simulink model "slau3"  (Simulink 9.1)
settings: Solver=ode45  StartTime=0.0  StopTime=5.0  RelTol=1e-3  EnableMultiTasking=on
settings Model: Creator=pustovskix.2018  LastModifiedBy=bukova.2018
settings DataIOCC: LimitDataPoints=on  SignalLoggingSaveFormat=ModelDataLogs
settings OptimizationCC: ExpressionDepthLimit=2147483647
settings DebuggingCC: SolverPrmCheckMsg=warning  FcnCallInpInsideContextMsg=warning  StateNameClashWarn=warning
settings GRTTargetCC: GeneratePreprocessorConditionals=Disable all

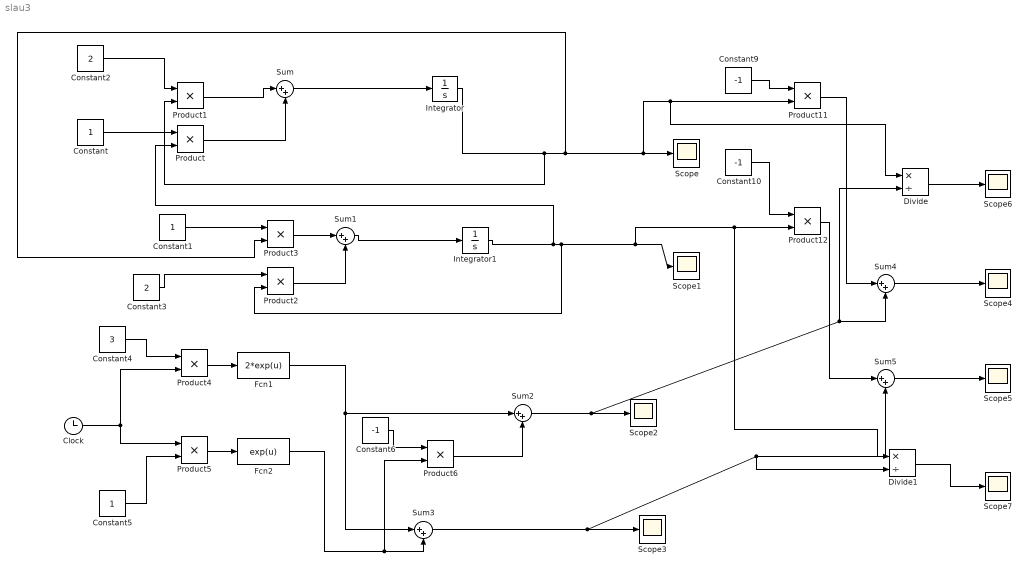
== system slau3 ==
  Clock : Clock
  Constant : Constant
  Constant1 : Constant
  Constant10 : Constant  Value=-1
  Constant2 : Constant  Value=2
  Constant3 : Constant  Value=2
  Constant4 : Constant  Value=3
  Constant5 : Constant
  Constant6 : Constant  Value=-1
  Constant9 : Constant  Value=-1
  Divide : Product  Inputs=*/
  Divide1 : Product  Inputs=*/
  Fcn1 : Fcn  Expr=2*exp(u)
  Fcn2 : Fcn  Expr=exp(u)
  Integrator : Integrator  InitialCondition=1
  Integrator1 : Integrator  InitialCondition=3
  Product{,1..6,11..12} (9 alike) : Product  RndMeth=Zero
  Scope{,1..7} (8 alike) : Scope
  Sum{,1..5} (6 alike) : Sum  Inputs=|++
  wires:
  Integrator1/1 -> Product2/2, Scope1/1, Divide1/1, Product12/2, Product/2
  Integrator/1 -> Product3/2, Scope/1, Divide/1, Product11/2, Product1/2
  Sum/1 -> Integrator/1
  Sum1/1 -> Integrator1/1
  Constant3/1 -> Product2/1
  Constant1/1 -> Product3/1
  Constant2/1 -> Product1/1
  Constant/1 -> Product/1
  Product1/1 -> Sum/1
  Product/1 -> Sum/2
  Product3/1 -> Sum1/1
  Product2/1 -> Sum1/2
  Clock/1 -> Product4/2, Product5/1
  Constant4/1 -> Product4/1
  Product4/1 -> Fcn1/1
  Constant10/1 -> Product12/1
  Constant9/1 -> Product11/1
  Product11/1 -> Sum4/1
  Product12/1 -> Sum5/1
  Sum5/1 -> Scope5/1
  Sum4/1 -> Scope4/1
  Sum2/1 -> Scope2/1, Divide/2, Sum4/2
  Sum3/1 -> Scope3/1, Divide1/2, Sum5/2
  Product5/1 -> Fcn2/1
  Constant5/1 -> Product5/2
  Fcn1/1 -> Sum3/1, Sum2/1
  Fcn2/1 -> Sum3/2, Product6/2
  Constant6/1 -> Product6/1
  Product6/1 -> Sum2/2
  Divide/1 -> Scope6/1
  Divide1/1 -> Scope7/1
